simulink model "ErmittlungderAPs"  (R2016a)
settings: Solver=VariableStepAuto  SolverMode=SingleTasking  StartTime=0.0  StopTime=500.0  RelTol=1e-3
values from neighbouring files (symbols this model uses):
  c = [0.005,1.53,0.5,0.18,121,27.9,198,2.36,5.74,11.35,16.1,201]    [Regerlung_einer_WEA.m]
  d_b = 2000    [Regerlung_einer_WEA.m]
  d_s = 6215000    [Moddel4DOF_onlylin.m]    (also in Regerlung_einer_WEA.m)
  d_t = 7000    [Regerlung_einer_WEA.m]
  J_g = 5025347    [Moddel4DOF_onlylin.m]    (also in Regerlung_einer_WEA.m = 534)
  J_r = 38759227    [Moddel4DOF_onlylin.m]    (also in Regerlung_einer_WEA.m)
  k_b = 40000    [Regerlung_einer_WEA.m]
  k_s = 867637000    [Moddel4DOF_onlylin.m]    (also in Regerlung_einer_WEA.m)
  k_t = 1981900    [Regerlung_einer_WEA.m]
  m_b = 4435    [Regerlung_einer_WEA.m]
  m_t = 436865    [Regerlung_einer_WEA.m]
  N = 3    [Moddel4DOF_onlylin.m]    (also in Regerlung_einer_WEA.m)
  n_g_inv = 1/n_g    (= 0.0103092783505)    [Regerlung_einer_WEA.m]
  R = 63    [Moddel4DOF_onlylin.m]    (also in Regerlung_einer_WEA.m)
  T_g_c = [0,0,0,43093.5,43093.5,43093.5]    [Regerlung_einer_WEA.m]
  theta_c = [0,0,0,4,15,22]*pi/180    [Regerlung_einer_WEA.m]
  v_c = [8.0,10.0,11.0,14.0,18.0,25.0]    [Regerlung_einer_WEA.m]    (also in testinterpolation.m = [9,9.5,10,11,14,15,18,25])
undefined symbols (not defined in the file or in its folder): F_t_c, i
settings Model: Creator=pasca  LastModifiedBy=pasca
settings DebuggingCC: SFUnexpectedBacktrackingDiag=error  SFNoUnconditionalDefaultTransitionDiag=error
settings GRTTargetCC: TargetLangStandard=C99 (ISO)  GeneratePreprocessorConditionals=Use local settings
settings ConfigComp: CovMetricSettings=dwe  CovHtmlReporting=off  CovSaveCumulativeToWorkspaceVar=off  CovSaveSingleToWorkspaceVar=off  CovExternalEMLEnable=on

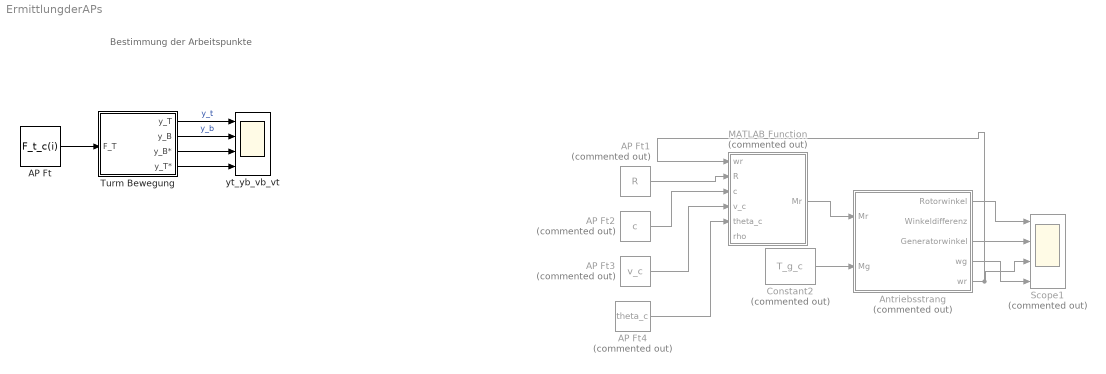
== system ErmittlungderAPs ==
  note: Bestimmung der Arbeitspunkte
  " Antriebsstrang" : Subsystem  Commented=on
  AP Ft : Constant  Value=F_t_c(i)
  AP Ft1 : Constant  Commented=on  Value=R
  AP Ft2 : Constant  Commented=on  Value=c
  AP Ft3 : Constant  Commented=on  Value=v_c
  AP Ft4 : Constant  Commented=on  Value=theta_c
  Constant2 : Constant  Commented=on  Value=T_g_c  VectorParams1D=off
  MATLAB Function : MATLAB Function  Commented=on  TreatAsAtomicUnit=on
  Scope1 : Scope  Commented=on  NumInputPorts=4
  Turm Bewegung : Subsystem
  yt_yb_vb_vt : Scope  NumInputPorts=4
  wires:
  AP Ft/1 -> Turm Bewegung/1(F_T)
  Turm Bewegung/1(y_T) -> yt_yb_vb_vt/1  "y_t"
  Turm Bewegung/2(y_B) -> yt_yb_vb_vt/2  "y_b"
  Turm Bewegung/3(y_B*) -> yt_yb_vb_vt/3
  Turm Bewegung/4(y_T*) -> yt_yb_vb_vt/4
  " Antriebsstrang"/3(Generatorwinkel) -> Scope1/2
  " Antriebsstrang"/1(Rotorwinkel) -> Scope1/1
  " Antriebsstrang"/4(wg) -> Scope1/4
  " Antriebsstrang"/5(wr) -> MATLAB Function/1(wr), Scope1/3
  Constant2/1 -> " Antriebsstrang"/2(Mg)
  MATLAB Function/1(Mr) -> " Antriebsstrang"/1(Mr)
  AP Ft1/1 -> MATLAB Function/2(R)
  AP Ft2/1 -> MATLAB Function/3(c)
  AP Ft3/1 -> MATLAB Function/4(v_c)
  AP Ft4/1 -> MATLAB Function/5(theta_c)

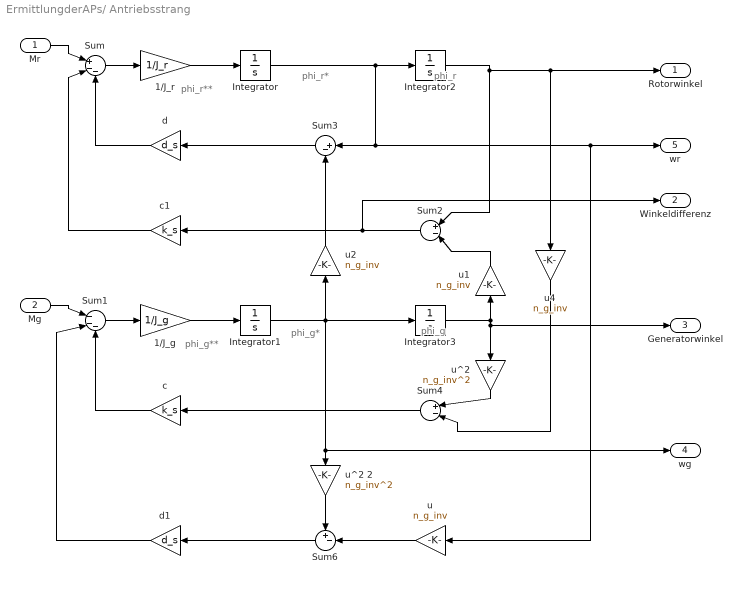
== system ErmittlungderAPs/ Antriebsstrang ==
  note: phi_g
  note: phi_r
  note: phi_g*
  note: phi_r*
  note: phi_g**
  note: phi_r**
  Mr : Inport
  Mg : Inport  Port=2
  1/J_g : Gain  Gain=1/J_g
  1/J_r : Gain  Gain=1/J_r
  Integrator{,1..3} (4 alike) : Integrator
  Sum : Sum  Inputs=|+--
  Sum1 : Sum  Inputs=|---
  Sum2 : Sum  Inputs=|+-|
  Sum3 : Sum  Inputs=|+-
  Sum4 : Sum  Inputs=|+-|
  Sum6 : Sum  Inputs=+-|
  c : Gain  Gain=k_s
  c1 : Gain  Gain=k_s
  d : Gain  Gain=d_s
  d1 : Gain  Gain=d_s
  u{,1..2,4} (4 alike) : Gain  Gain=n_g_inv
  u^2 : Gain  Gain=n_g_inv^2
  u^2 2 : Gain  Gain=n_g_inv^2
  Rotorwinkel : Outport
  Winkeldifferenz : Outport  Port=2
  Generatorwinkel : Outport  Port=3
  wg : Outport  Port=4
  wr : Outport  Port=5
  wires:
  Sum/1 -> 1/J_r/1
  Mg/1 -> Sum1/1
  Mr/1 -> Sum/1
  Sum1/1 -> 1/J_g/1
  1/J_r/1 -> Integrator/1
  1/J_g/1 -> Integrator1/1
  Integrator/1 -> Sum3/1, wr/1, u/1, Integrator2/1
  Integrator1/1 -> u2/1, Integrator3/1, u^2 2/1, wg/1
  Integrator2/1 -> Rotorwinkel/1, u4/1, Sum2/1
  Sum2/1 -> c1/1, Winkeldifferenz/1
  Integrator3/1 -> Generatorwinkel/1, u^2/1, u1/1
  u1/1 -> Sum2/2
  c1/1 -> Sum/2
  u2/1 -> Sum3/2
  Sum3/1 -> d/1
  d/1 -> Sum/3
  u4/1 -> Sum4/2
  u^2/1 -> Sum4/1
  Sum4/1 -> c/1
  c/1 -> Sum1/3
  u/1 -> Sum6/2
  u^2 2/1 -> Sum6/1
  d1/1 -> Sum1/2
  Sum6/1 -> d1/1

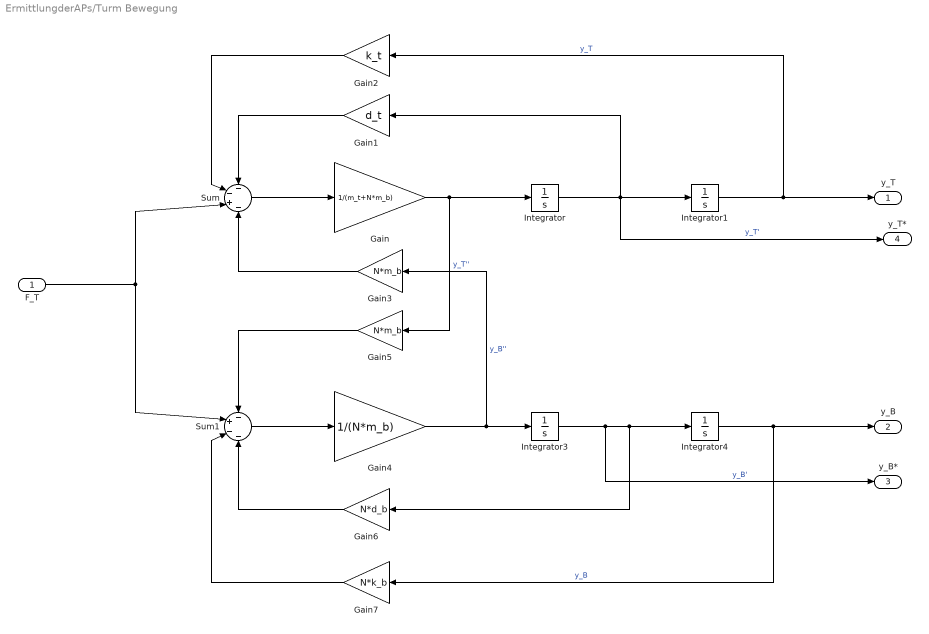
== system ErmittlungderAPs/Turm Bewegung ==
  F_T : Inport
  Gain : Gain  Gain=1/(m_t+N*m_b)
  Gain1 : Gain  Gain=d_t
  Gain2 : Gain  Gain=k_t
  Gain3 : Gain  Gain=N*m_b
  Gain4 : Gain  Gain=1/(N*m_b)
  Gain5 : Gain  Gain=N*m_b
  Gain6 : Gain  Gain=N*d_b
  Gain7 : Gain  Gain=N*k_b
  Integrator{,1,3..4} (4 alike) : Integrator
  Sum : Sum  Inputs=--+-
  Sum1 : Sum  Inputs=-+--
  y_T : Outport
  y_B : Outport  Port=2
  y_B* : Outport  Port=3
  y_T* : Outport  Port=4
  wires:
  Integrator1/1 -> Gain2/1, y_T/1  "y_T"
  Integrator/1 -> y_T*/1, Gain1/1, Integrator1/1  "y_T'"
  Integrator4/1 -> y_B/1, Gain7/1  "y_B"
  Integrator3/1 -> y_B*/1, Gain6/1, Integrator4/1  "y_B'"
  Gain/1 -> Gain5/1, Integrator/1  "y_T''"
  F_T/1 -> Sum1/2, Sum/3
  Gain1/1 -> Sum/1
  Sum/1 -> Gain/1
  Gain2/1 -> Sum/2
  Gain3/1 -> Sum/4
  Gain4/1 -> Gain3/1, Integrator3/1  "y_B''"
  Sum1/1 -> Gain4/1
  Gain5/1 -> Sum1/1
  Gain6/1 -> Sum1/4
  Gain7/1 -> Sum1/3

== matlab function ErmittlungderAPs/MATLAB Function ==
  data: wr input; Mr output; R input; c input; v_c input; theta_c input; rho input
function Mr = fcn(wr,R,c,v_c,theta_c,rho)
lambda_local=(wr*R)/v_c;
lambda_i_local = (1/(lambda_local+(0.08*theta_c)))-(0.035/(c(11)+(c(12)*theta_c^3)));
f_0_local = c(1)*(1+c(2)*(theta_c+c(3))^(1/2));
f_1_local = c(4)/lambda_local;
f_2_local = ((c(5)*lambda_i_local)-(c(6)*theta_c)-(c(7)*theta_c^c(8))-c(9));
f_3_local = exp(-c(10)*lambda_i_local);
CM_tilde_local =f_0_local+f_1_local*f_2_local*f_3_local;
CM_local = CM_tilde_local*(1+sign(CM_tilde_local))/2;
Mr=0.5*rho*pi*R^3*v_c^2*CM_local*n_g_inv;
